simulink model "PX03s"  (R2015b)
settings: Solver=VariableStepAuto  StartTime=0.0  StopTime=3  RelTol=1e-3
libraries: fl_lib x14, nesl_utility x3
settings Model: Creator=xmax1946  LastModifiedBy=xmax1946

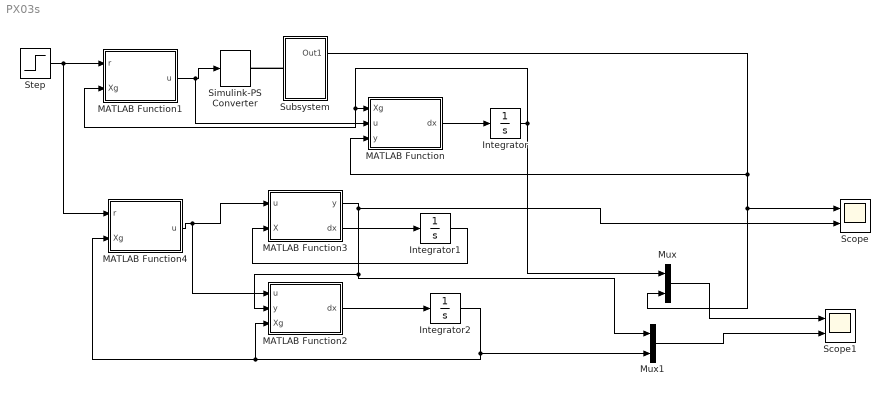
== system PX03s ==
  Integrator : Integrator  InitialCondition=[1]
  Integrator1 : Integrator  InitialCondition=[0]  IgnoreLimit=on
  Integrator2 : Integrator  InitialCondition=[1]
  MATLAB Function : MATLAB Function  TreatAsAtomicUnit=on
  MATLAB Function1 : MATLAB Function  TreatAsAtomicUnit=on
  MATLAB Function2 : MATLAB Function  TreatAsAtomicUnit=on
  MATLAB Function3 : MATLAB Function  TreatAsAtomicUnit=on
  MATLAB Function4 : MATLAB Function  TreatAsAtomicUnit=on
  Mux : Mux  Inputs=2
  Mux1 : Mux  Inputs=2
  Scope : Scope  NumInputPorts=2
  Scope1 : Scope  NumInputPorts=2
  Simulink-PS Converter : nesl_utility/Simulink-PS Converter  PhysicalDomain=network_engine_domain  SubClassName=ps_input  LeftPortType=input  RightPortType=output  PseudoPeriodic=off  Frequencies=[]  NoiseDistribution=none  NoiseParameters=[]  Unit=1  AffineConversion=off  InputFiltering=off  SimscapeFilterOrder=1  InputFilterTimeConstant=0.001  UdotUserProvided=1
  Step : Step  SampleTime=0
  Subsystem : Subsystem
  wires:
  MATLAB Function/1(dx) -> Integrator/1
  MATLAB Function1/1(u) -> MATLAB Function/2(u), Simulink-PS Converter/1
  MATLAB Function4/1(u) -> MATLAB Function2/1(u), MATLAB Function3/1(u)
  MATLAB Function2/1(dx) -> Integrator2/1
  MATLAB Function3/2(dx) -> Integrator1/1
  Integrator1/1 -> MATLAB Function3/2(X)
  MATLAB Function3/1(y) -> Scope/2, Mux1/1, MATLAB Function2/2(y)
  Mux/1 -> Scope1/1
  Mux1/1 -> Scope1/2
  Subsystem/1(Out1) -> Mux/2, Scope/1, MATLAB Function/3(y)
  Integrator/1 -> MATLAB Function1/2(Xg), MATLAB Function/1(Xg), Mux/1
  Integrator2/1 -> MATLAB Function4/2(Xg), MATLAB Function2/3(Xg), Mux1/2
  Step/1 -> MATLAB Function4/1(r), MATLAB Function1/1(r)
  connections:
  Subsystem/LConn1 -- Simulink-PS Converter/RConn1

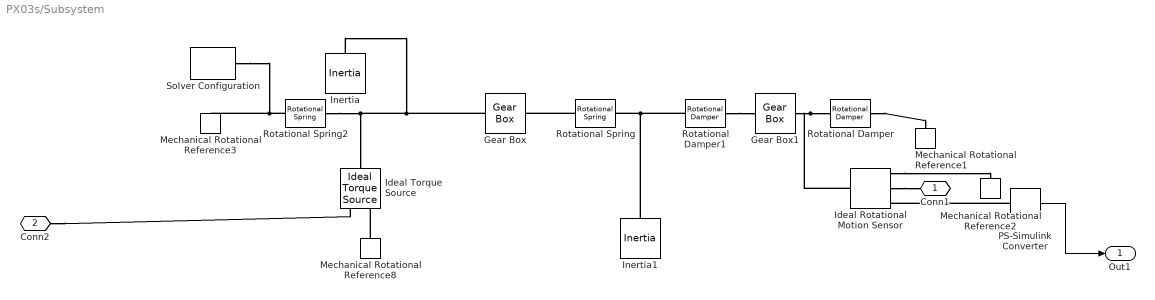
== system PX03s/Subsystem ==
  Gear Box : fl_lib/Mechanical/Mechanisms/Gear Box  ratio=10  t_in_specify=off  t_in_priority=None  t_in=0 N*m  t_out_specify=off  t_out_priority=None  t_out=0 N*m
  Gear Box1 : fl_lib/Mechanical/Mechanisms/Gear Box  ratio=10  t_in_specify=off  t_in_priority=None  t_in=0 N*m  t_out_specify=off  t_out_priority=None  t_out=0 N*m
  Ideal Rotational Motion Sensor : fl_lib/Mechanical/Mechanical Sensors/Ideal Rotational Motion Sensor  offset=0 rad
  Ideal Torque Source : fl_lib/Mechanical/Mechanical Sources/Ideal Torque Source
  Inertia : fl_lib/Mechanical/Rotational Elements/Inertia  inertia=0.000001 kg*m^2  w_specify=off  w_priority=None  w=0 rad/s  t_specify=off  t_priority=None  t=0 N*m
  Inertia1 : fl_lib/Mechanical/Rotational Elements/Inertia  inertia=0.000001 kg*m^2  w_specify=off  w_priority=None  w=0 rad/s  t_specify=off  t_priority=None  t=0 N*m
  Mechanical Rotational Reference{1..3,8} (4 alike) : fl_lib/Mechanical/Rotational Elements/Mechanical Rotational Reference
  PS-Simulink Converter : nesl_utility/PS-Simulink Converter  PhysicalDomain=network_engine_domain  SubClassName=ps_output  LeftPortType=input  RightPortType=output  PseudoPeriodic=off  Frequencies=[]  Unit=1  AffineConversion=off
  Rotational Damper : fl_lib/Mechanical/Rotational Elements/Rotational Damper  D=200 N*m/(rad/s)  w_specify=off  w_priority=None  w=0 rad/s  t_specify=off  t_priority=None  t=0 N*m
  Rotational Damper1 : fl_lib/Mechanical/Rotational Elements/Rotational Damper  D=3 N*m/(rad/s)  w_specify=off  w_priority=None  w=0 rad/s  t_specify=off  t_priority=None  t=0 N*m
  Rotational Spring : fl_lib/Mechanical/Rotational Elements/Rotational Spring  spr_rate=2 N*m/rad  w_specify=off  w_priority=None  w=0 rad/s  t_specify=off  t_priority=None  t=0 N*m  phi_specify=off  phi_priority=None  phi=0 rad
  Rotational Spring2 : fl_lib/Mechanical/Rotational Elements/Rotational Spring  spr_rate=1/10 N*m/rad  w_specify=off  w_priority=None  w=0 rad/s  t_specify=off  t_priority=None  t=0 N*m  phi_specify=off  phi_priority=None  phi=0 rad
  Solver Configuration : nesl_utility/Solver Configuration  PhysicalDomain=network_engine_domain  SubClassName=solver  LeftPortType=input  RightPortType=generic  Accelerate=off  Tones=[]  Harmonics=[]  SimulateNoise=off  Profile=off  UseLocalSampling=off  EnableSwitchedLinearOptims=on  FrequencyDomain=off  UseCCode=off  RelTol=0.001  AbsTol=1e-06  MinStep=1e-09  ToWorkspace=off  RevertToSquareIcSolve=off  NumHomotopyIterations=100  PhasorMode=off  PhasorModeNumHarmonics=1  DoDC=off  ResidualTolerance=1e-09  UseLocalSolver=off  LocalSolverChoice=NE_TRAPEZOIDAL_ADVANCER  LocalSolverSampleTime=0.001  DoFixedCost=off  MaxNonlinIter=3  MaxModeIter=2  LinearAlgebra=Sparse  DelaysMemoryBudget=1024  AutomaticFiltering=on  FilteringTimeConstant=0.001
  Conn1 : PMIOPort  Port=1  Side=Right
  Conn2 : PMIOPort  Port=2  Side=Left
  Out1 : Outport
  wires:
  PS-Simulink Converter/1 -> Out1/1
  connections:
  Rotational Spring/LConn1 -- Gear Box/RConn1
  Rotational Damper/RConn1 -- Mechanical Rotational Reference1/LConn1
  Ideal Rotational Motion Sensor/RConn1 -- Mechanical Rotational Reference2/LConn1
  Gear Box/LConn1 -- Rotational Spring2/RConn1 -- Ideal Torque Source/LConn1 -- Inertia/LConn1
  Rotational Spring2/LConn1 -- Solver Configuration/RConn1 -- Mechanical Rotational Reference3/LConn1
  Gear Box1/RConn1 -- Ideal Rotational Motion Sensor/LConn1 -- Rotational Damper/LConn1
  PS-Simulink Converter/LConn1 -- Ideal Rotational Motion Sensor/RConn3
  Rotational Damper1/LConn1 -- Inertia1/LConn1 -- Rotational Spring/RConn1
  Rotational Damper1/RConn1 -- Gear Box1/LConn1
  Conn2/RConn1 -- Ideal Torque Source/RConn1
  Mechanical Rotational Reference8/LConn1 -- Ideal Torque Source/RConn2
  Ideal Rotational Motion Sensor/RConn2 -- Conn1/RConn1

== matlab function PX03s/MATLAB Function1 ==
  data: r input; u output; Xg input
function u = fcn(r,Xg)
K=[29/15];
u=r-K*Xg;

== matlab function PX03s/MATLAB Function ==
  data: dx output; Xg input; u input; y input
function dx  = fss(Xg,u,y)
A=[-25/18];
B=[5/6];
C=[1/10];
L=[415/9];
dx=A*Xg+B*u+L*(y-C*Xg);

== matlab function PX03s/MATLAB Function2 ==
  data: u input; y input; Xg input; dx output
function dx  = fcn(u,y,Xg)
A=[-25/18];
B=[5/6];
C=[1/10];
L=[415/9];
dx=A*Xg+B*u+L*(y-C*Xg);

== matlab function PX03s/MATLAB Function3 ==
  data: u input; y output; X input; dx output
function [y,dx] = fcn(u,X)
A=[-25/18];
B=[5/6];
C=[1/10];
dx=A*X+B*u;
y=C*X;

== matlab function PX03s/MATLAB Function4 ==
  data: r input; u output; Xg input
function u = fcn(r,Xg)
K=[29/15];
u=r-K*Xg;
